simulink subsystem "Thruster_Magnitude"  (R2022b)
settings: Solver=VariableStepAuto  StartTime=0.0  StopTime=10.0  RelTol=1e-3
settings Model: Creator=hayden  LastModifiedBy=hollis
settings ModelReferenceCC: EnableRefExpFcnMdlSchedulingChecks=on

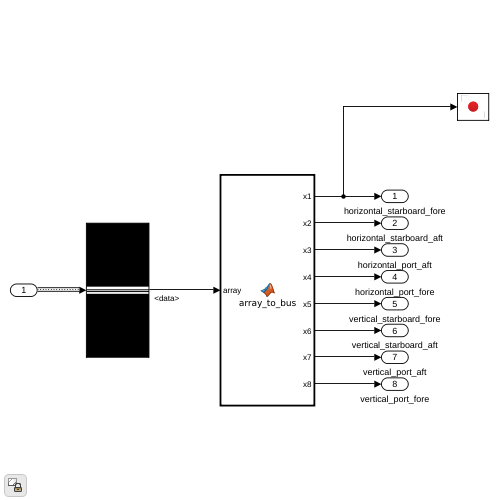
[thumbnail: Simulink's stored preview of the top-level diagram]
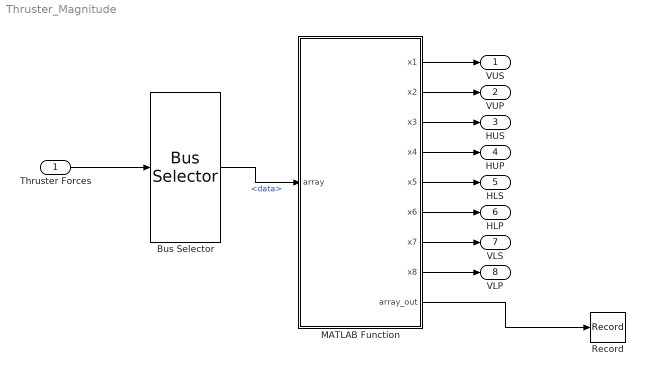
== system Thruster_Magnitude ==
  Thruster Forces : Inport
  Bus Selector : BusSelector  OutputSignals=data
  MATLAB Function : MATLAB Function  TreatAsAtomicUnit=on
  Record : Record  FileSettingsInternal="{\"entries\":[{\"content\":{\"excelSettings\":{\"content\":{},\"type\":\"Streamout.ExcelSettings\"}},\"type\":\"Streamout.FileSettingStorage\",\"uuid\":\"c4f85216-62a6-4c7c-80c1-9999ceb0d5cc\"}],\"packageUris\":[\"http://schema.mathworks.com/mf0/streamout_blocks/R2020a\"],\"version\":\"1.0\"}"  Layout=[1 1]  SignalsInternal="{\"entries\":[{\"content\":{\"signals\":[{\"content\":{\"blockPath\":[\"Thruster_Magnitude/Record\"],\"channel\":[],\"dimensions\":[1,8],\"domain\":\"Thruster_Magnitude/Record\",\"hasChildren\":true,\"lineColor\":\"#edb120\",\"plots\":[],\"port\":1,\"sid\":[],\"signalID\":332,\"signalName\":\"MATLAB Function:9\"},\"type\":\"RecordBlkView.Signal\",\"uuid\":\"3a90f5e8-568a-4ed5-a849-75e6847f0cdb\"},{\"content\":{\"blockPath\":[\"Thruster_Magnitude/Record\"],\"channel\":[1,1],\"dimensions\":[1,8],\"domain\":\"Thruster_Magnitude/Record\",\"lineColor\":\"#7e2f8e\",\"parentID\":332,\"plots\":[1],\"port\":1,\"sid\":[],\"signalID\":333,\"signalName\":\"MATLAB Function:9\"},\"type\":\"RecordBlkView.Signal\",\"uuid\":\"beaa4f09-a0c4-47fd-bd84-415099834234\"},{\"content\":{\"blockPath\":[\"Thruster_Magnitude/Record\"],\"channel\":[1,2],\"dimensions\":[1,8],\"domain\":\"Thruster_Magnitude/Record\",\"lineColor\":\"#7e2f8e\",\"parentID\":332,\"plots\":[1],\"port\":1,\"sid\":[],\"signalID\":334,\"signalName\":\"MATLAB Function:9\"},\"type\":\"RecordBlkView.Signal\",\"uuid\":\"375c414b-fe38-46ae-b8b2-37f7bfb761dc\"},{\"content\":{\"blockPath\":[\"Thruster_Magnitude/Record\"],\"channel\":[1,3],\"dimensions\":[1,8],\"domain\":\"Thruster_Magnitude/Record\",\"lineColor\":\"#77ac30\",\"parentID\":332,\"plots\":[1],\"port\":1,\"sid\":[],\"signalID\":335,\"signalName\":\"MATLAB Function:9\"},\"type\":\"RecordBlkView.Signal\",\"uuid\":\"9d27270b-4c4d-450b-a120-228dfcd428bc\"},{\"content\":{\"blockPath\":[\"Thruster_Magnitude/Record\"],\"channel\":[1,4],\"dimensions\":[1,8],\"domain\":\"Thruster_Magnitude/Record\",\"lineColor\":\"#4dbeee\",\"parentID\":332,\"plots\":[1],\"port\":1,\"sid\":[],\"signalID\":336,\"signalName\":\"MATLAB Function:9\"},\"type\":\"RecordBlkView.Signal\",\"uuid\":\"68feee60-1350-4b67-b87b-7693f4990d0c\"},{\"content\":{\"blockPath\":[\"Thruster_Magnitude/Record\"],\"channel\":[1,5],\"dimensions\":[1,8],\"domain\":\"Thruster_Magnitude/Record\",\"lineColor\":\"#a2142f\",\"parentID\":332,\"plots\":[1],\"port\":1,\"sid\":[],\"signalID\":337,\"signalName\":\"MATLAB Function:9\"},\"type\":\"RecordBlkView.Signal\",\"uuid\":\"f0bb4909-5272-46c3-9ed4-759dfa1c2878\"},{\"content\":{\"blockPath\":[\"Thruster_Magnitude/Record\"],\"channel\":[1,6],\"dimensions\":[1,8],\"domain\":\"Thruster_Magnitude/Record\",\"lineColor\":\"#139fff\",\"parentID\":332,\"plots\":[1],\"port\":1,\"sid\":[],\"signalID\":338,\"signalName\":\"MATLAB Function:9\"},\"type\":\"RecordBlkView.Signal\",\"uuid\":\"1cb7f022-26bc-45e4-a4d5-d600aed2fdf1\"},{\"content\":{\"blockPath\":[\"Thruster_Magnitude/Record\"],\"channel\":[1,7],\"dimensions\":[1,8],\"domain\":\"Thruster_Magnitude/Record\",\"lineColor\":\"#ff6929\",\"parentID\":332,\"plots\":[1],\"port\":1,\"sid\":[],\"signalID\":339,\"signalName\":\"MATLAB Function:9\"},\"type\":\"RecordBlkView.Signal\",\"uuid\":\"f9afa5d9-a0b6-46e4-827b-97b62fb72892\"},{\"content\":{\"blockPath\":[\"Thruster_Magnitude/Record\"],\"channel\":[1,8],\"dimensions\":[1,8],\"domain\":\"Thruster_Magnitude/Record\",\"lineColor\":\"#b746ff\",\"parentID\":332,\"plots\":[1],\"port\":1,\"sid\":[],\"signalID\":340,\"signalName\":\"MATLAB Function:9\"},\"type\":\"RecordBlkView.Signal\",\"uuid\":\"a077ca82-29b6-412f-80ff-a10a871b972f\"}]},\"type\":\"RecordBlkView.InputSignals\",\"uuid\":\"53731d8b-1cd3-471b-bae9-b732aa776438\"}],\"packageUris\":[\"http://schema.mathworks.com/mf0/streamout_blocks/R2020a\"],\"version\":\"1.0\"}"  VisualizationBindings="{\"sparklinesplugin\":{\"info\":[{\"bindingParametersList\":[],\"subplotID\":1}]}}"
  VUS : Outport
  VUP : Outport  Port=2
  HUS : Outport  Port=3
  HUP : Outport  Port=4
  HLS : Outport  Port=5
  HLP : Outport  Port=6
  VLS : Outport  Port=7
  VLP : Outport  Port=8
  wires:
  Bus Selector/1 -> MATLAB Function/1(array)  "<data>"
  MATLAB Function/1(x1) -> VUS/1
  MATLAB Function/2(x2) -> VUP/1
  MATLAB Function/3(x3) -> HUS/1
  MATLAB Function/4(x4) -> HUP/1
  MATLAB Function/5(x5) -> HLS/1
  MATLAB Function/6(x6) -> HLP/1
  MATLAB Function/7(x7) -> VLS/1
  MATLAB Function/8(x8) -> VLP/1
  Thruster Forces/1 -> Bus Selector/1
  MATLAB Function/9(array_out) -> Record/1

== matlab function Thruster_Magnitude/MATLAB Function ==
  data: array input; x1 output; x2 output; x3 output; x4 output; x5 output; x6 output; x7 output; x8 output; array_out output
function [x1,x2,x3,x4,x5,x6,x7,x8, array_out] = array_to_bus(array)

    x1 = array(1);
    x2 = array(2);
    x3 = array(3);
    x4 = array(4);
    x5 = array(5);
    x6 = array(6);
    x7 = array(7);
    x8 = array(8);

    array_out = [x1,x2,x3,x4,x5,x6,x7,x8];
end
